simulink model "auv_model"  (R2020a)
settings: Solver=VariableStepAuto  StartTime=0.0  StopTime=10.0  RelTol=1e-3
settings Model: Creator=mluser  LastModifiedBy=mluser

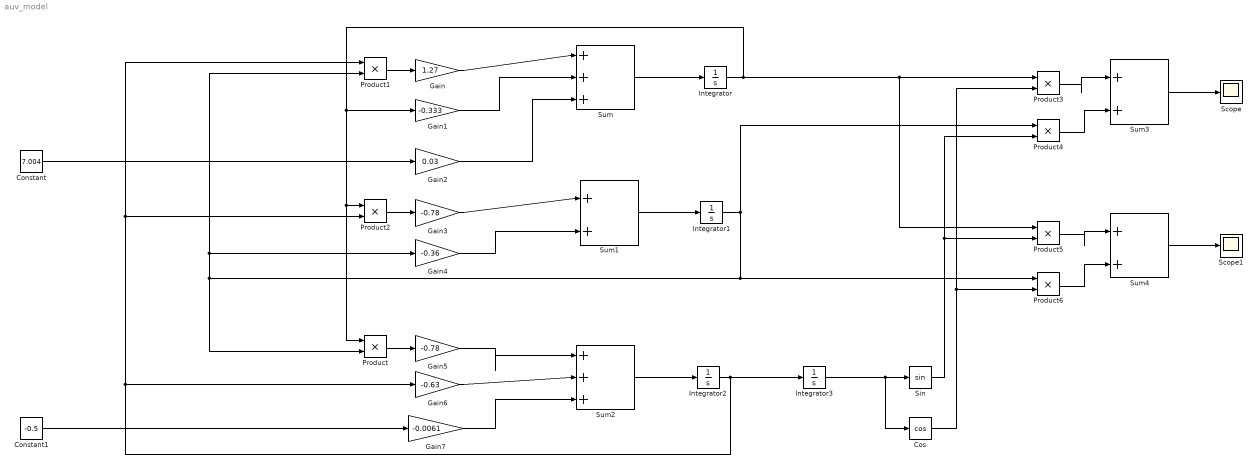
== system auv_model ==
  Constant : Constant  Value=7.004
  Constant1 : Constant  Value=-0.5
  Cos : Trigonometry  Operator=cos
  Gain : Gain  Gain=1.27
  Gain1 : Gain  Gain=-0.333
  Gain2 : Gain  Gain=0.03
  Gain3 : Gain  Gain=-0.78
  Gain4 : Gain  Gain=-0.36
  Gain5 : Gain  Gain=-0.78
  Gain6 : Gain  Gain=-0.63
  Gain7 : Gain  Gain=-0.0061
  Integrator{,1..3} (4 alike) : Integrator
  Product{,1..6} (7 alike) : Product
  Scope : Scope
  Scope1 : Scope
  Sin : Trigonometry
  Sum : Sum  Inputs=|+++
  Sum1 : Sum  Inputs=|++
  Sum2 : Sum  Inputs=|+++
  Sum3 : Sum  Inputs=|++
  Sum4 : Sum  Inputs=|++
  wires:
  Sum/1 -> Integrator/1
  Gain1/1 -> Sum/2
  Gain/1 -> Sum/1
  Gain2/1 -> Sum/3
  Sum2/1 -> Integrator2/1
  Gain5/1 -> Sum2/1
  Gain6/1 -> Sum2/2
  Gain7/1 -> Sum2/3
  Integrator/1 -> Product5/1, Product3/1, Product/1, Product2/1, Gain1/1
  Product1/1 -> Gain/1
  Gain3/1 -> Sum1/1
  Integrator1/1 -> Product4/1, Product6/1, Product1/2, Gain4/1, Product/2
  Sum1/1 -> Integrator1/1
  Gain4/1 -> Sum1/2
  Product2/1 -> Gain3/1
  Product/1 -> Gain5/1
  Integrator2/1 -> Integrator3/1, Product2/2, Product1/1, Gain6/1
  Constant/1 -> Gain2/1
  Constant1/1 -> Gain7/1
  Integrator3/1 -> Cos/1, Sin/1
  Cos/1 -> Product6/2, Product3/2
  Sin/1 -> Product4/2, Product5/2
  Product3/1 -> Sum3/1
  Product4/1 -> Sum3/2
  Product5/1 -> Sum4/1
  Product6/1 -> Sum4/2
  Sum3/1 -> Scope/1
  Sum4/1 -> Scope1/1
